simulink model "pendu_vesc"  (R2018b)
settings: Solver=FixedStepAuto  StartTime=0.0  StopTime=inf  RelTol=1e-3  EnableMultiTasking=on
libraries: peGeneralControl x3, cm_custom x2, simulink x1
settings Model: SimulationMode=external  Creator=Ng Wee Shen  LastModifiedBy=Ng Wee Shen
settings SolverCC: PositivePriorityOrder=on  AutoInsertRateTranBlk=on
settings OptimizationCC: EnhancedBackFolding=on  PassReuseOutputArgsAs=Individual arguments  MaxStackSize=64  OptimizeBlockOrder=speed  DifferentSizesBufferReuse=on
settings DebuggingCC: TimeAdjustmentMsg=warning  SingleTaskRateTransMsg=warning  ParameterTunabilityLossMsg=error  SFcnCompatibilityMsg=warning
settings HardwareCC: ProdBitPerPointer=32  ProdBitPerSizeT=32  ProdBitPerPtrDiffT=32  ProdLargestAtomicInteger=Long  ProdLargestAtomicFloat=Double  ProdWordSize=32  ProdHWDeviceType=ARM Compatible->ARM Cortex
settings SFSimCC: MATLABDynamicMemAlloc=off
settings RTWCC: SystemTargetFile=ert.tlc  HardwareBoard=Raspberry Pi  TLCOptions="-aInlineSetEventsForThisBaseRateFcn=TLC_FALSE -aSuppressMultiTaskScheduler=TLC_FALSE  -aRateBasedStepFcn=0"  TemplateMakefile=ert_default_tmf  Toolchain=GNU GCC Raspberry Pi  BuildConfiguration=Specify  IncludeHyperlinkInReport=on  TargetLang=C++
settings CodeAppCC: ForceParamTrailComments=on  IgnoreCustomStorageClasses=off  OperatorAnnotations=on  SimulinkDataObjDesc=on  SFDataObjDesc=on  InsertBlockDesc=on
settings ERTTargetCC: TargetLangStandard=C++03 (ISO)  SupportContinuousTime=on  SupportVariableSizeSignals=on  ExtMode=on  ExtModeMexArgs='192.168.0.173' 1 17725

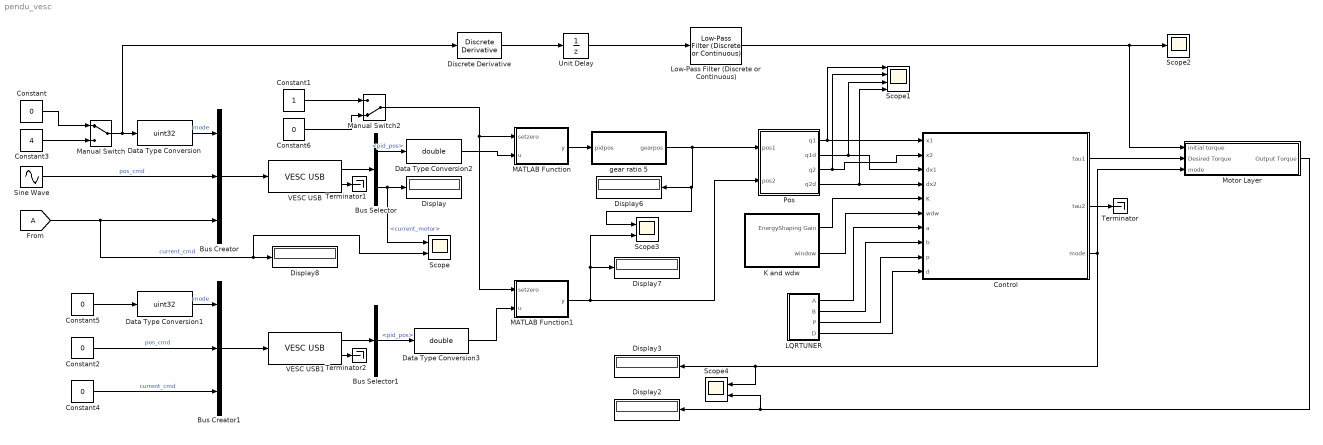
== system pendu_vesc ==
  Bus Creator : BusCreator  Inputs=3
  Bus Creator1 : BusCreator  Inputs=3
  Bus Selector : BusSelector  OutputSignals=pid_pos,current_motor
  Bus Selector1 : BusSelector  OutputSignals=pid_pos
  Constant{,2,4..6} (5 alike) : Constant  Value=0
  Constant1 : Constant
  Constant3 : Constant  Value=4
  Control : MATLAB Function  TreatAsAtomicUnit=on
  Data Type Conversion : DataTypeConversion  OutDataTypeStr=uint32
  Data Type Conversion1 : DataTypeConversion  OutDataTypeStr=uint32
  Data Type Conversion2 : DataTypeConversion  OutDataTypeStr=double
  Data Type Conversion3 : DataTypeConversion  OutDataTypeStr=double
  Discrete Derivative : simulink/Discrete/Discrete Derivative  gainval=1.0  ICPrevScaledInput=0.0  OutMin=[]  OutMax=[]  OutDataType=fixdt(1, 16)  OutScaling=2^-10  DoSatur=off
  Display{,2..3,6..8} (6 alike) : Display
  K and wdw : Subsystem
  LQRTUNER : Subsystem
  Low-Pass Filter (Discrete or Continuous) : peGeneralControl/Low-Pass Filter (Discrete or Continuous)  K=-1  T=0.025  B=0.05  A=-0.05  Ts=-1
  MATLAB Function : MATLAB Function  TreatAsAtomicUnit=on
  MATLAB Function1 : MATLAB Function  TreatAsAtomicUnit=on
  Manual Switch : ManualSwitch
  Manual Switch2 : ManualSwitch  CurrentSetting=0
  Motor Layer : Subsystem
  Pos : Subsystem
  Scope : Scope  NumInputPorts=2
  Scope1 : Scope  NumInputPorts=4
  Scope2 : Scope
  Scope3 : Scope  NumInputPorts=2
  Scope4 : Scope  NumInputPorts=2
  Sine Wave : Sin  Amplitude=150  Bias=10  SampleTime=0
  Terminator : Terminator
  Terminator1 : Terminator
  Terminator2 : Terminator
  Unit Delay : UnitDelay  SampleTime=-1
  VESC USB : cm_custom/VESC USB  PAR_VESC_DEV='/dev/USB_VESC2'  POS_KP=0.03  POS_KI=0  POS_KD=0.0004  POS_KD_FIL=0.2  POS_DIV=1  CURR_MAX=6  CURR_MIN=-6  CURR_IN_MAX=99  CURR_IN_MIN=-60  CURR_ABS_MAX=130  PAR_SMPLT=0.001
      settings: SourceProductName=cm custom
  VESC USB1 : cm_custom/VESC USB  PAR_VESC_DEV='/dev/USB_VESC1'  POS_KP=0.001  POS_KI=0  POS_KD=0.001  POS_KD_FIL=0.2  POS_DIV=1  CURR_MAX=20  CURR_MIN=-20  CURR_IN_MAX=20  CURR_IN_MIN=-20  CURR_ABS_MAX=20  PAR_SMPLT=0.001
      settings: SourceProductName=cm custom
  gear ratio 5 : Subsystem
  wires:
  Bus Creator/1 -> VESC USB/1
  VESC USB/1 -> Bus Selector/1
  VESC USB/2 -> Terminator1/1
  Data Type Conversion/1 -> Bus Creator/1  "mode"
  Bus Selector/2 -> Display/1, Scope/1  "<current_motor>"
  Bus Selector/1 -> Data Type Conversion2/1  "<pid_pos>"
  Constant3/1 -> Manual Switch/2
  Constant/1 -> Manual Switch/1
  Sine Wave/1 -> Bus Creator/2  "pos_cmd"
  [A] -> Scope/2, Display8/1, Bus Creator/3  "current_cmd"
  Constant4/1 -> Bus Creator1/3  "current_cmd"
  Data Type Conversion1/1 -> Bus Creator1/1  "mode"
  Constant2/1 -> Bus Creator1/2  "pos_cmd"
  Bus Creator1/1 -> VESC USB1/1
  Constant5/1 -> Data Type Conversion1/1
  Bus Selector1/1 -> Data Type Conversion3/1  "<pid_pos>"
  VESC USB1/1 -> Bus Selector1/1
  VESC USB1/2 -> Terminator2/1
  Pos/1(q1) -> Scope1/1, Control/1(x1)
  Pos/2(q1d) -> Scope1/3, Control/3(dx1)
  Pos/4(q2d) -> Scope1/4, Control/4(dx2)
  K and wdw/1(EnergyShaping Gain) -> Control/5(K)
  K and wdw/2(window) -> Control/6(wdw)
  LQRTUNER/3(P) -> Control/9(p)
  LQRTUNER/4(D) -> Control/10(d)
  LQRTUNER/2(B) -> Control/8(b)
  LQRTUNER/1(A) -> Control/7(a)
  Control/2(tau2) -> Terminator/1
  Motor Layer/1(Output Torque) -> Scope4/2, Display2/1
  Control/3(mode) -> Motor Layer/3(" mode "), Scope4/1, Display3/1
  Data Type Conversion2/1 -> MATLAB Function/2(u)
  MATLAB Function1/1(y) -> Pos/2(pos2), Display7/1, Scope3/2
  Data Type Conversion3/1 -> MATLAB Function1/2(u)
  Constant1/1 -> Manual Switch2/1
  Constant6/1 -> Manual Switch2/2
  Manual Switch2/1 -> MATLAB Function1/1(setzero), MATLAB Function/1(setzero)
  Pos/3(q2) -> Scope1/2, Control/2(x2)
  MATLAB Function/1(y) -> gear ratio 5/1(pidpos)
  gear ratio 5/1(gearpos) -> Pos/1(pos1), Scope3/1, Display6/1
  Manual Switch/1 -> Discrete Derivative/1, Data Type Conversion/1
  Control/1(tau1) -> Motor Layer/2(Desired Torque)
  Discrete Derivative/1 -> Unit Delay/1
  Unit Delay/1 -> Low-Pass Filter (Discrete or Continuous)/1
  Low-Pass Filter (Discrete or Continuous)/1 -> Motor Layer/1(initial torque), Scope2/1

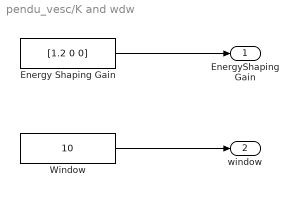
== system pendu_vesc/K and wdw ==
  Energy Shaping Gain : Constant  Value=[1.2 0 0]
  Window : Constant  Value=10
  EnergyShaping Gain : Outport
  window : Outport  Port=2
  wires:
  Energy Shaping Gain/1 -> EnergyShaping Gain/1
  Window/1 -> window/1

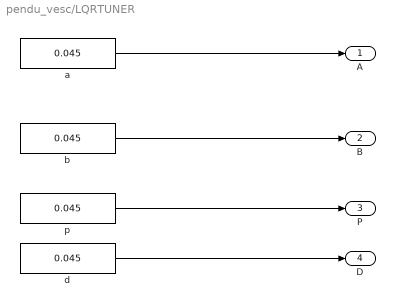
== system pendu_vesc/LQRTUNER ==
  a : Constant  Value=0.045
  b : Constant  Value=0.045
  d : Constant  Value=0.045
  p : Constant  Value=0.045
  A : Outport
  B : Outport  Port=2
  P : Outport  Port=3
  D : Outport  Port=4
  wires:
  p/1 -> P/1
  b/1 -> B/1
  d/1 -> D/1
  a/1 -> A/1

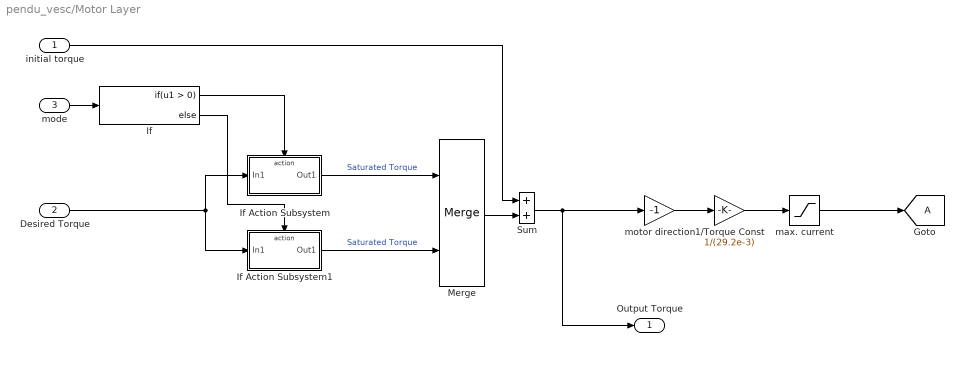
== system pendu_vesc/Motor Layer ==
  initial torque : Inport
  Desired Torque : Inport  Port=2
  " mode " : Inport  Port=3
  1/Torque Const : Gain  Gain=1/(29.2e-3)  OutDataTypeStr=Inherit: Same as input
  If : If
  If Action Subsystem : Subsystem  TreatAsAtomicUnit=on
  If Action Subsystem1 : Subsystem  TreatAsAtomicUnit=on
  Merge : Merge
  Sum : Sum
  max. current : Saturate  UpperLimit=3  LowerLimit=-3  LinearizeAsGain=off
  motor direction : Gain  Gain=-1  OutDataTypeStr=Inherit: Same as input
  Output Torque : Outport
  tag scope: A=global
  wires:
  motor direction/1 -> 1/Torque Const/1
  1/Torque Const/1 -> max. current/1
  max. current/1 -> [A]
  " mode "/1 -> If/1
  Desired Torque/1 -> If Action Subsystem/1(In1), If Action Subsystem1/1(In1)
  If Action Subsystem/1(Out1) -> Merge/1  "Saturated Torque"
  If Action Subsystem1/1(Out1) -> Merge/2  "Saturated Torque"
  If/1 -> If Action Subsystem/Action
  If/2 -> If Action Subsystem1/Action
  Merge/1 -> Sum/2
  Sum/1 -> Output Torque/1, motor direction/1
  initial torque/1 -> Sum/1

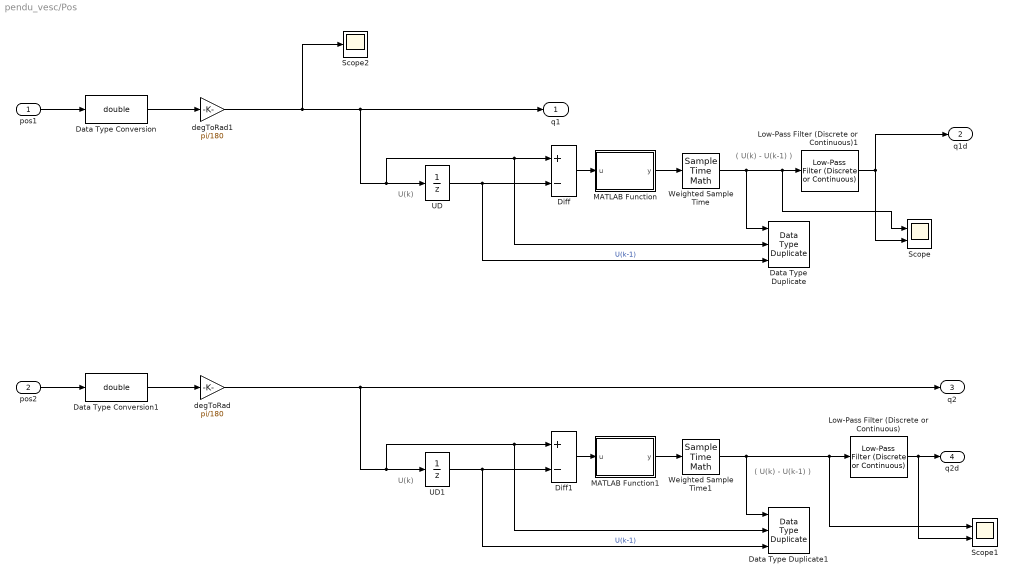
== system pendu_vesc/Pos ==
  note: ( U(k) - U(k-1) )
  note: U(k)
  note: U(k)
  note: ( U(k) - U(k-1) )
  pos1 : Inport
  pos2 : Inport  Port=2
  Data Type Duplicate : DataTypeDuplicate  DisableCoverage=on  NumInputPorts=3
  Data Type Duplicate1 : DataTypeDuplicate  DisableCoverage=on  NumInputPorts=3
  Data Type Conversion : DataTypeConversion  OutDataTypeStr=double
  Data Type Conversion1 : DataTypeConversion  OutDataTypeStr=double
  Diff : Sum  Description=Add in CPU  Inputs=+-
  Diff1 : Sum  Description=Add in CPU  Inputs=+-
  Low-Pass Filter (Discrete or Continuous) : peGeneralControl/Low-Pass Filter (Discrete or Continuous)  K=1  T=0.01  B=inf  A=-inf  Ts=-1
  Low-Pass Filter (Discrete or Continuous)1 : peGeneralControl/Low-Pass Filter (Discrete or Continuous)  K=1  T=0.01  B=inf  A=-inf  Ts=-1
  MATLAB Function : MATLAB Function  TreatAsAtomicUnit=on
  MATLAB Function1 : MATLAB Function  TreatAsAtomicUnit=on
  Scope : Scope  NumInputPorts=2
  Scope1 : Scope  NumInputPorts=2
  Scope2 : Scope
  UD : UnitDelay  Description=Store in Global RAM  DisableCoverage=on  SampleTime=-1
  UD1 : UnitDelay  Description=Store in Global RAM  DisableCoverage=on  SampleTime=-1
  Weighted Sample Time : SampleTimeMath  TsampMathOp=/
  Weighted Sample Time1 : SampleTimeMath  TsampMathOp=/
  degToRad : Gain  Gain=pi/180
  degToRad1 : Gain  Gain=pi/180
  q1 : Outport
  q1d : Outport  Port=2
  q2 : Outport  Port=3
  q2d : Outport  Port=4
  wires:
  pos2/1 -> Data Type Conversion1/1
  pos1/1 -> Data Type Conversion/1
  Data Type Conversion1/1 -> degToRad/1
  Data Type Conversion/1 -> degToRad1/1
  Diff/1 -> MATLAB Function/1(u)
  UD/1 -> Diff/2, Data Type Duplicate/3  "U(k-1)"
  MATLAB Function/1(y) -> Weighted Sample Time/1
  Weighted Sample Time/1 -> Data Type Duplicate/1, Scope/1, Low-Pass Filter (Discrete or Continuous)1/1
  UD1/1 -> Diff1/2, Data Type Duplicate1/3  "U(k-1)"
  Diff1/1 -> MATLAB Function1/1(u)
  MATLAB Function1/1(y) -> Weighted Sample Time1/1
  Weighted Sample Time1/1 -> Data Type Duplicate1/1, Scope1/1, Low-Pass Filter (Discrete or Continuous)/1
  degToRad1/1 -> Scope2/1, q1/1, UD/1, Diff/1, Data Type Duplicate/2
  Low-Pass Filter (Discrete or Continuous)/1 -> Scope1/2, q2d/1
  Low-Pass Filter (Discrete or Continuous)1/1 -> Scope/2, q1d/1
  degToRad/1 -> q2/1, UD1/1, Diff1/1, Data Type Duplicate1/2

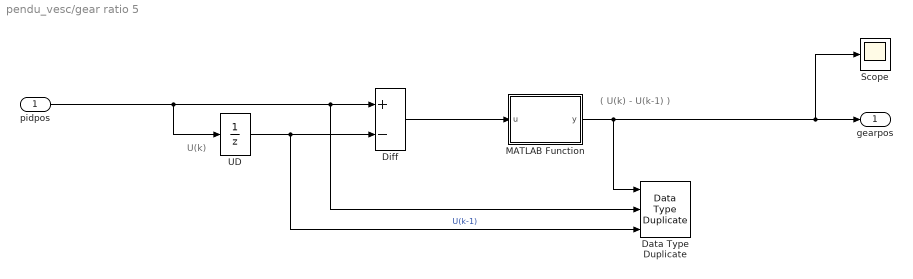
== system pendu_vesc/gear ratio 5 ==
  note: ( U(k) - U(k-1) )
  note: U(k)
  pidpos : Inport
  Data Type Duplicate : DataTypeDuplicate  DisableCoverage=on  NumInputPorts=3
  Diff : Sum  Description=Add in CPU  Inputs=+-
  MATLAB Function : MATLAB Function  TreatAsAtomicUnit=on
  Scope : Scope
  UD : UnitDelay  Description=Store in Global RAM  DisableCoverage=on  SampleTime=-1
  gearpos : Outport
  wires:
  UD/1 -> Diff/2, Data Type Duplicate/3  "U(k-1)"
  pidpos/1 -> UD/1, Diff/1, Data Type Duplicate/2
  MATLAB Function/1(y) -> Data Type Duplicate/1, Scope/1, gearpos/1
  Diff/1 -> MATLAB Function/1(u)

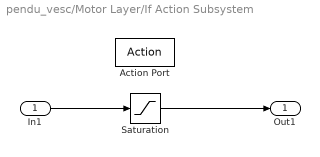
== system pendu_vesc/Motor Layer/If Action Subsystem ==
  In1 : Inport
  Action Port : ActionPort  ActionType=then
  Saturation : Saturate  UpperLimit=0.055  LowerLimit=-0.055
  Out1 : Outport
  wires:
  In1/1 -> Saturation/1
  Saturation/1 -> Out1/1

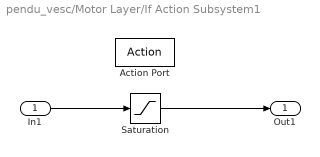
== system pendu_vesc/Motor Layer/If Action Subsystem1 ==
  In1 : Inport
  Action Port : ActionPort  ActionType=else
  Saturation : Saturate  UpperLimit=0.035  LowerLimit=-0.035
  Out1 : Outport
  wires:
  In1/1 -> Saturation/1
  Saturation/1 -> Out1/1

== matlab function pendu_vesc/MATLAB Function ==
  data: setzero input; u input; y output
function y = fcn(setzero,u)

persistent initpos
if isempty(initpos)
    initpos = 0;
end

if setzero
    initpos = u + 0;
end


y = u - initpos;
y = y - 360*floor(y/360);

== matlab function pendu_vesc/Control ==
  data: x1 input; tau1 output; x2 input; dx1 input; dx2 input; K input; wdw input; a input; b input; p input; d input; tau2 output; mode output
function [tau1,tau2,mode] = EnergyShaping_w_LQR(x1,x2,dx1,dx2,K,wdw,a,b,p,d)
% Match the setup in simulation
x = [x1;x2;dx1;dx2]; 

persistent model;
if isempty(model)
    model = Model();
end

%%%%
q  = x(1:2,:);
qd = x(3:4,:);

[tau,mode] = acrobotControlLaw_LQR(x,wdw,a,b,p,d);

if isempty(tau) % if LQR control law is not applicable, 
                %    then using Energy Shaping approach
    mode = 0;
    g  = model.g;
    %
    l1 = model.l1; lc1 = model.lc1; l2 = model.l2; lc2 = model.lc2;
    m1 = model.m1; m2 = model.m2;
    I1 = model.I1; I2 = model.I2;
    b1 = model.b1; b2 = model.b2;

    %%%%
    q  = x(1:2,:);
    qd = x(3:4,:);

    %%%%
    c = cos(q(1:2,:));  s = sin(q(1:2,:));  c12 = cos(q(1,:)+q(2,:));
    
    [M,~] = ManipulatorEquation(model, x);
    %%%% energy shaping
    E_des = m1.*g.* lc1 + m2.*g.*(l1+lc2);

    KE = 0.5*qd.'*M*qd;
    PE = -m1*g*lc1*c(1) - m2*g*(l1*c(1)+lc2*c12);
    E = KE + PE;

    E_tilda = E_des - E;

%     ke = 1;    %0.75  %5   %0.05;
%     kd = 0*ke/10;  %25   %ke/15;
%     ks = 0*kd/5;   %8   %kd/10;
    ke = K(1);
    kd = K(2)*ke;
    ks = K(3)*kd;
    
    q(1) = q(1) - 2*pi*floor(q(1)./(2*pi));
    d_tilda = pi-q(1);
    s_tilda = 0-qd(1);
    
    % P-saturation
    PD = d_tilda*kd + s_tilda*ks;
    if abs(PD) > 1
        PD = 1 * sign(PD);
    end
    
    tau = [(ke.*E_tilda.*qd(1)+PD); 0]; 
    %tau = [(0); 0]; 
    
end
tau=(18/90)*tau;
tau1 = tau(1);

tau2 = tau(2);
end

== matlab function pendu_vesc/MATLAB Function1 ==
  data: setzero input; u input; y output
function y = fcn(setzero,u)

persistent initpos
if isempty(initpos)
    initpos = 0;
end

if setzero
    initpos = u + 0;
end


y = u - initpos;
y = y - 360*floor(y/360);

== matlab function pendu_vesc/Pos/MATLAB Function ==
  data: u input; y output
function y = fcn(u)

u_rev = (u >= 0)*(2*pi - u) + (u < 0)*(2*pi + u);

if abs(u_rev) > abs(u)
   y = u;
else
   y = (u < 0)*u_rev - (u >= 0)*u_rev;
end

== matlab function pendu_vesc/Pos/MATLAB Function1 ==
  data: u input; y output
function y = fcn(u)

u_rev = (u >= 0)*(2*pi - u) + (u < 0)*(2*pi + u);

if abs(u_rev) > abs(u)
   y = u;
else
   y = (u < 0)*u_rev - (u >= 0)*u_rev;
end

== matlab function pendu_vesc/gear ratio 5/MATLAB Function ==
  data: u input; y output
function y = fcn(u)

persistent pos1
if isempty(pos1)
    pos1 = 0;
end

u_rev = (u >= 0)*(360 - u) + (u < 0)*(360 + u);
if abs(u_rev) < abs(u)
   u = (u < 0)*u_rev - (u >= 0)*u_rev;
end

u = u/5;
pos1 = pos1 + u;
pos1 = mod((pos1),360);
y = pos1;

end
